simulink model "NGradosLibertadRetoSS"  (R2022a)
settings: Solver=VariableStepAuto  StartTime=0.0  StopTime=1000  RelTol=1e-3
settings Model: Creator=aafo_  LastModifiedBy=aafo_

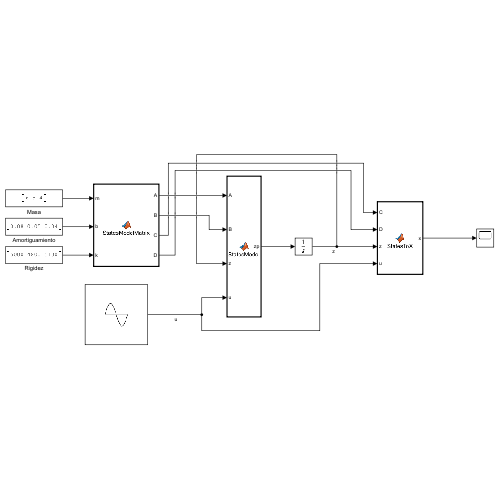
[thumbnail: Simulink's stored preview of the top-level diagram]
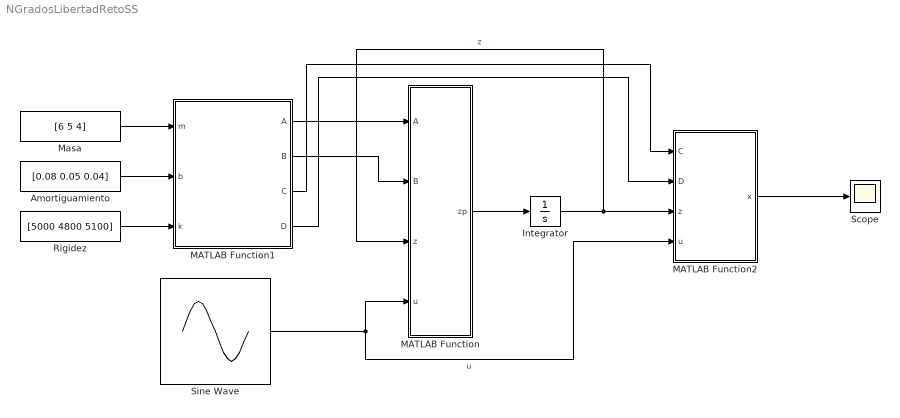
== system NGradosLibertadRetoSS ==
  Amortiguamiento : Constant  Value=[0.08 0.05 0.04]
  Integrator : Integrator  InitialCondition=[0 0 0 0 0 0]'
  MATLAB Function : MATLAB Function  TreatAsAtomicUnit=on
  MATLAB Function1 : MATLAB Function  TreatAsAtomicUnit=on
  MATLAB Function2 : MATLAB Function  TreatAsAtomicUnit=on
  Masa : Constant  Value=[6 5 4]
  Rigidez : Constant  Value=[5000 4800 5100]
  Scope : Scope
  Sine Wave : Sin  Frequency=14.6176  SampleTime=0
  wires:
  Amortiguamiento/1 -> MATLAB Function1/2(b)
  Rigidez/1 -> MATLAB Function1/3(k)
  Masa/1 -> MATLAB Function1/1(m)
  MATLAB Function1/1(A) -> MATLAB Function/1(A)
  MATLAB Function1/2(B) -> MATLAB Function/2(B)
  MATLAB Function/1(zp) -> Integrator/1
  Integrator/1 -> MATLAB Function/3(z), MATLAB Function2/3(z)  "z"
  MATLAB Function1/3(C) -> MATLAB Function2/1(C)
  MATLAB Function1/4(D) -> MATLAB Function2/2(D)
  Sine Wave/1 -> MATLAB Function/4(u), MATLAB Function2/4(u)  "u"
  MATLAB Function2/1(x) -> Scope/1

== matlab function NGradosLibertadRetoSS/MATLAB Function1 ==
  data: m input; A output; b input; k input; B output; C output; D output
function [A, B, C, D] = StatesModelMatrix(m, b, k)

n = length(m);

M = zeros(n);

for i = 1:n
    M(i,i) = m(i);

end

B_ = zeros(n);

for i = 1:n
    for j = 1:n
        if j == i+1
            B_(i,j) = -b(i+1);
        elseif j == i-1
            B_(i,j) = -b(i);
        elseif i==j
            if  i == n && j == n
                B_(i,j) = b(n);
            else
                B_(i,j) = b(i)+b(i+1);
            end
        else
            B_(i,j) = 0;
        end
    end
end

K = zeros(n);

for i = 1:n
    for j = 1:n
        if j == i+1
            K(i,j) = -k(i+1);
        elseif j == i-1
            K(i,j) = -k(i);
        elseif i==j
            if  i == n && j == n
                K(i,j) = k(n);
            else
                K(i,j) = k(i)+k(i+1);
            end
        else
            K(i,j) = 0;
        end
    end
end


A = [zeros(n) eye(n); -inv(M)*K -inv(M)*B_];
B = [zeros(n,1); -ones(n, 1)];
C = [eye(n) zeros(n)];
D = zeros(n,1);

== matlab function NGradosLibertadRetoSS/MATLAB Function ==
  data: A input; B input; z input; u input; zp output
function zp = StatesModel(A , B, z, u)

zp = A*z+B*u;

== matlab function NGradosLibertadRetoSS/MATLAB Function2 ==
  data: C input; D input; z input; x output; u input
function x = StatesToX(C, D, z, u)

x = C*z + D*u;
